simulink model "selector2D"  (Simulink 7.3)
settings: Solver=ode3  StartTime=0.0  StopTime=10.0  FixedStep=1  RelTol=1e-3
settings Model: Creator=hnine  LastModifiedBy=hnine
settings OptimizationCC: InitFltsAndDblsToZero=on
settings DebuggingCC: SaveWithParameterizedLinksMsg=none
settings GRTTargetCC: TargetFcnLib=ansi_tfl_tmw.mat

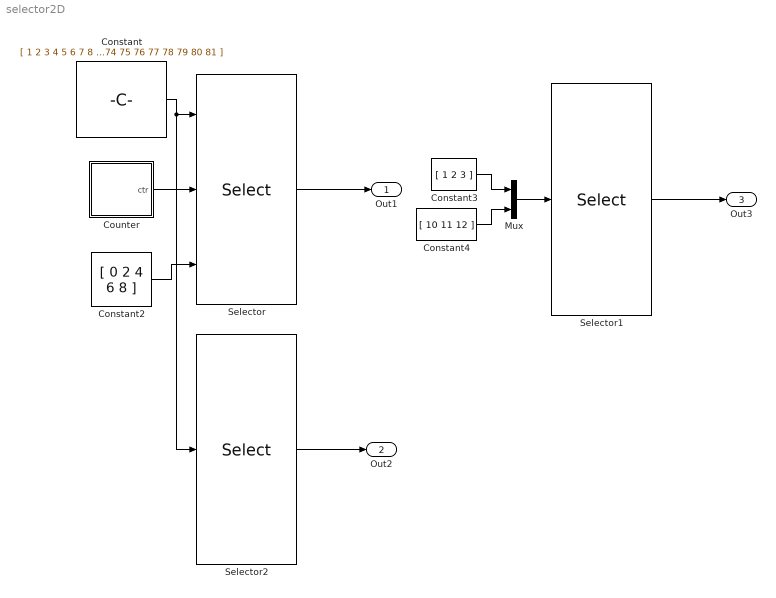
== system selector2D ==
  Constant : Constant  Value=[ 1 2 3 4 5 6 7 8 9 ; 10 11 12 13 14 15 16 17 18 ; 19 20 21 22 23 24 25 26 27 ; 28 29 30 31 32 33 34 35 36 ; 37 38 39 40 41 42 43 44 45 ; 46 47 48 49 50 51 52 53 54 ; 55 56 57 58 59 60 61 62 63 ; 64 65 66 67 68 69 70 71 72 ; 73 74 75 76 77 78 79 80 81 ]  VectorParams1D=off  OutDataType=sfix(16)  OutScaling=2^0
  Constant2 : Constant  Value=[ 0 2 4 6 8 ]  VectorParams1D=off  OutDataType=sfix(16)  OutScaling=2^0
  Constant3 : Constant  Value=[ 1 2 3 ]  VectorParams1D=off  OutDataType=sfix(16)  OutScaling=2^0
  Constant4 : Constant  Value="[ 10 11 12  ]"  VectorParams1D=off  OutDataType=sfix(16)  OutScaling=2^0
  Counter : Stateflow chart
  Mux : Mux  Inputs=2
  Selector : Selector  NumberOfDimensions=2  IndexMode=Zero-based  InputPortWidth=3  IndexOptions=Starting index (port),Index vector (port)  Indices=[1 3],2  OutputSizes=3,5
  Selector1 : Selector  IndexOptions=Index vector (dialog)  Indices=[1 3 4 5]  OutputSizes=3
  Selector2 : Selector  NumberOfDimensions=2  InputPortWidth=3  IndexOptions=Starting index (dialog),Select all  Indices=2,2  OutputSizes=1,5
  Out1 : Outport  OutDataType=sfix(16)  OutScaling=2^0
  Out2 : Outport  Port=2  OutDataType=sfix(16)  OutScaling=2^0
  Out3 : Outport  Port=3  OutDataType=sfix(16)  OutScaling=2^0
  wires:
  Counter/1(ctr) -> Selector/2
  Constant2/1 -> Selector/3
  Constant3/1 -> Mux/1
  Constant4/1 -> Mux/2
  Constant/1 -> Selector/1, Selector2/1
  Mux/1 -> Selector1/1
  Selector/1 -> Out1/1
  Selector2/1 -> Out2/1
  Selector1/1 -> Out3/1

== stateflow chart Counter ==
  state s1
  (default) -> s1
  s1 -> s1 [order 1] : [ctr < 4] / ctr = ctr+1;
  s1 -> s1 [order 2] : [ctr >= 4] / ctr = 0;
  data: ctr output double =1
